simulink model "Path_Sim"  (R2018a)
settings: Solver=VariableStepAuto  StartTime=0.0  StopTime=10.0  RelTol=1e-3
libraries: dspindex x1
settings Model: Creator=chrros005  LastModifiedBy=chrros005

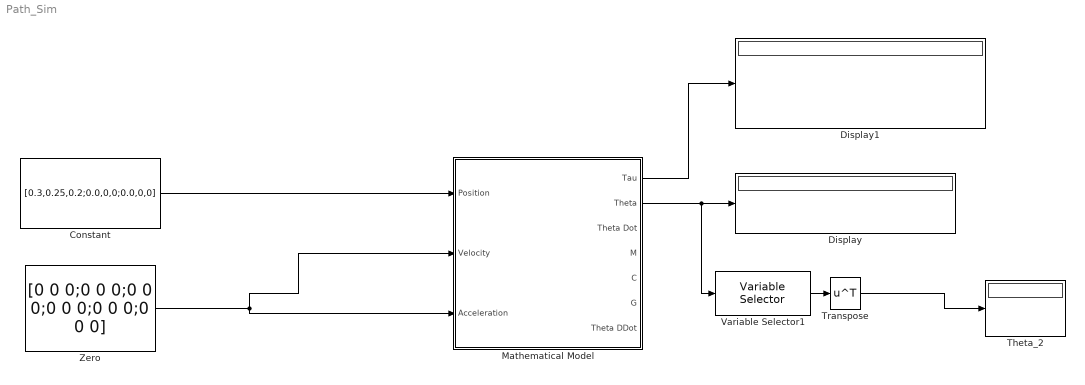
== system Path_Sim ==
  Constant : Constant  Value=[0.3,0.25,0.2;0.0,0,0;0.0,0,0]
  Display : Display
  Display1 : Display
  "Mathematical Model " : Subsystem  TreatAsAtomicUnit=on
  Theta_2 : Display
  Transpose : Math  Operator=transpose  SaturateOnIntegerOverflow=on
  Variable Selector1 : dspindex/Variable Selector  NumInputs=1  rowsOrCols=Rows  IdxMode=Fixed  Elements=2  ZerOneIdxMode=One-based  errmode=Clip Index  FillMode=on  FillValues=0
  Zero : Constant  Value=[0 0 0;0 0 0;0 0 0;0 0 0;0 0 0;0 0 0]
  wires:
  Constant/1 -> "Mathematical Model "/1(Position)
  Zero/1 -> "Mathematical Model "/2(Velocity), "Mathematical Model "/3(Acceleration)
  "Mathematical Model "/2(Theta) -> Variable Selector1/1, Display/1
  Variable Selector1/1 -> Transpose/1
  Transpose/1 -> Theta_2/1
  "Mathematical Model "/1(Tau) -> Display1/1

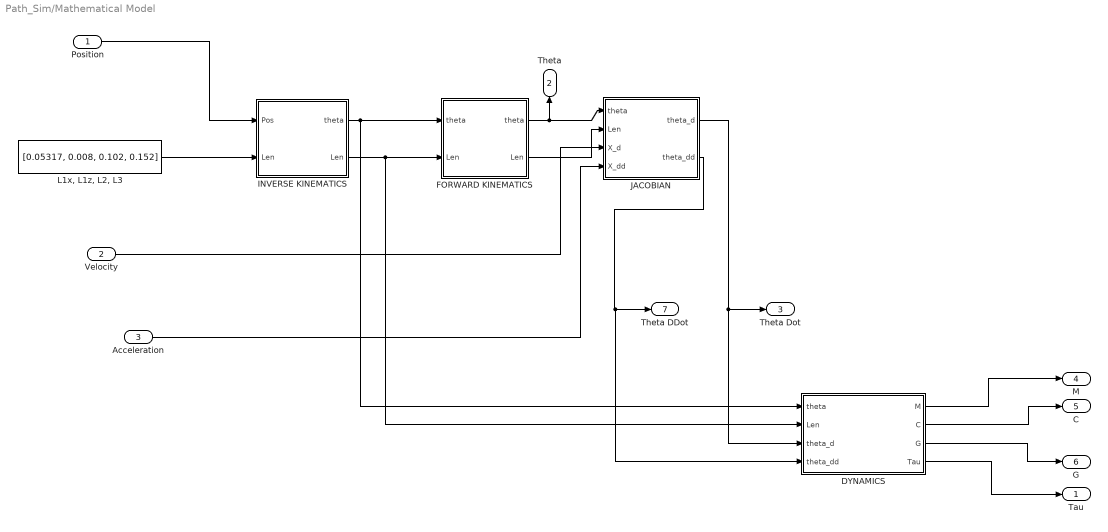
== system Path_Sim/Mathematical Model  ==
  Position : Inport
  Velocity : Inport  Port=2
  Acceleration : Inport  Port=3
  "DYNAMICS " : MATLAB Function  TreatAsAtomicUnit=on
  "FORWARD KINEMATICS " : MATLAB Function  TreatAsAtomicUnit=on
  "INVERSE KINEMATICS " : MATLAB Function  TreatAsAtomicUnit=on
  JACOBIAN : MATLAB Function  TreatAsAtomicUnit=on
  "L1x, L1z, L2, L3" : Constant  Value=[0.05317, 0.008, 0.102, 0.152]
  Tau : Outport
  Theta : Outport  Port=2
  Theta Dot : Outport  Port=3
  M : Outport  Port=4
  C : Outport  Port=5
  G : Outport  Port=6
  Theta DDot : Outport  Port=7
  wires:
  "INVERSE KINEMATICS "/1(theta) -> "FORWARD KINEMATICS "/1("theta "), "DYNAMICS "/1(theta)
  "FORWARD KINEMATICS "/2(Len) -> JACOBIAN/2(Len)
  "FORWARD KINEMATICS "/1(theta) -> JACOBIAN/1(theta), Theta/1
  JACOBIAN/2(theta_dd) -> Theta DDot/1, "DYNAMICS "/4(theta_dd)
  "L1x, L1z, L2, L3"/1 -> "INVERSE KINEMATICS "/2("Len ")
  "INVERSE KINEMATICS "/2(Len) -> "DYNAMICS "/2(Len), "FORWARD KINEMATICS "/2("Len ")
  "DYNAMICS "/4(Tau) -> Tau/1
  Acceleration/1 -> JACOBIAN/4(X_dd)
  Velocity/1 -> JACOBIAN/3(X_d)
  Position/1 -> "INVERSE KINEMATICS "/1(Pos)
  JACOBIAN/1(theta_d) -> Theta Dot/1, "DYNAMICS "/3(theta_d)
  "DYNAMICS "/1(M) -> M/1
  "DYNAMICS "/2(C) -> C/1
  "DYNAMICS "/3(G) -> G/1

== matlab function Path_Sim/Mathematical Model /FORWARD KINEMATICS  ==
  data: theta output; Len output; theta input; Len input
function [theta,Len]= FWD(theta, Len)
    
    s = size(theta);

    theta1 = theta(1,:);
    theta2 = theta(2,:);
    theta3 = theta(3,:);
   
    L1x = Len(1);
    L1z = Len(2);
    L2 = Len(3);
    L3 = Len(4); 
    

%     T = zeros(4,4,s(2));
%   
%     T = [ cos(theta2 + theta3)*cos(theta1), -sin(theta1), -sin(theta2 + theta3)*cos(theta1), cos(theta1)*(L1x + L3*cos(theta2 + theta3) + L2*cos(theta2));
%           cos(theta2 + theta3)*sin(theta1),  cos(theta1), -sin(theta2 + theta3)*sin(theta1), sin(theta1)*(L1x + L3*cos(theta2 + theta3) + L2*cos(theta2));
%                       sin(theta2 + theta3),            0,              cos(theta2 + theta3),               L1z + L3*sin(theta2 + theta3) + L2*sin(theta2);
%                                          0,            0,                                 0,                                                            1];

== matlab function Path_Sim/Mathematical Model /INVERSE KINEMATICS  ==
  data: Pos input; theta output; Len input; Len output
function [theta, Len] = INV(Pos, Len)

        s = size(Pos);

        x = zeros(1,s(2));
        y = zeros(1,s(2));
        z = zeros(1,s(2));

        theta1 = zeros(1,s(2));
        theta2 = zeros(1,s(2));
        theta3 = zeros(1,s(2));
        theta = zeros(3,s(2));
    
        x(:) = Pos(1,:);
        y(:) = Pos(2,:);
        z(:) = Pos(3,:);

        L1x = Len(1);
        L1z = Len(2);
        L2 = Len(3);
        L3 = Len(4);

        theta1(1,:) =  ( atan2(y(1,:),x(1,:)) );

        C3 = zeros(1,s(2));
        S3 = zeros(1,s(2));
        C3(1,:) = ( ( x(1,:) - L1x.*cos(theta1(1,:)) ).^2 + ( y(1,:) - L1x.*sin(theta1(1,:)) ).^2 + ( z(1,:) - L1z ).^2 - L2.^2 - L3.^2 )./( 2*L2*L3 );
        S3(1,:) = -sqrt(1 - C3(1,:).^2);

        theta2(1,:) =  ( atan2( z(1,:)-L1z, sqrt( (x(1,:)-L1x.*cos(theta1(1,:))).^2 + (y(1,:) - L1x.*sin(theta1(1,:))).^2 ) ) - atan2(L3.*S3(1,:), L2 + L3.*C3(1,:)) );

        theta3(1,:) =  ( atan2(S3(1,:), C3(1,:)) );

        theta = [theta1(1,:); theta2(1,:); theta3(1,:)];

== matlab function Path_Sim/Mathematical Model /JACOBIAN ==
  data: theta input; Len input; X_d input; theta_d output; theta_dd output; X_dd input
function [theta_d, theta_dd]= JAC(theta, Len, X_d, X_dd)

    s = size(theta);
    
    L1x = Len(1);
    L1z = Len(2);
    L2 = Len(3);
    L3 = Len(4);
        
    for i=1:s(2)

        theta1 = theta(1,i);
        theta2 = theta(2,i);
        theta3 = theta(3,i);
        
        J = zeros(6,3,s(2));

        J(:,:,i) = [-sin(theta1)*(L1x + L3*cos(theta2 + theta3) + L2*cos(theta2)), cos(theta1)*(L3*sin(theta2 + theta3) + L2*sin(theta2)), L3*sin(theta2 + theta3)*cos(theta1);
            cos(theta1)*(L1x + L3*cos(theta2 + theta3) + L2*cos(theta2)), sin(theta1)*(L3*sin(theta2 + theta3) + L2*sin(theta2)), L3*sin(theta2 + theta3)*sin(theta1);
                                                                 0,             - L3*cos(theta2 + theta3) - L2*cos(theta2),            -L3*cos(theta2 + theta3);
                                                                 0,                                           -sin(theta1),                        -sin(theta1);
                                                                 0,                                            cos(theta1),                         cos(theta1);
                                                                 1,                                                      0,                                   0]
        J_plus = zeros(3,6,s(2));
        J_plus(:,:,i) = [ -(2*sin(theta1)*(L1x + L3*cos(theta2 + theta3) + L2*cos(theta2)))/(L2^2*cos(2*theta2) + L3^2*cos(2*theta2 + 2*theta3) + L2^2 + L3^2 + 2*L1x^2 + 2*L2*L3*cos(2*theta2 + theta3) + 4*L3*L1x*cos(theta2 + theta3) + 2*L2*L3*cos(theta3) + 4*L2*L1x*cos(theta2) + 2), (2*cos(theta1)*(L1x + L3*cos(theta2 + theta3) + L2*cos(theta2)))/(L2^2*cos(2*theta2) + L3^2*cos(2*theta2 + 2*theta3) + L2^2 + L3^2 + 2*L1x^2 + 2*L2*L3*cos(2*theta2 + theta3) + 4*L3*L1x*cos(theta2 + theta3) + 2*L2*L3*cos(theta3) + 4*L2*L1x*cos(theta2) + 2),                                                                                                                                                                                 0,                                                                         0,                                                                        0, 1/((L2^2*cos(2*theta2))/2 + (L3^2*cos(2*theta2 + 2*theta3))/2 + L2^2/2 + L3^2/2 + L1x^2 + L2*L3*cos(2*theta2 + theta3) + 2*L3*L1x*cos(theta2 + theta3) + L2*L3*cos(theta3) + 2*L2*L1x*cos(theta2) + 1);
                                                                                                                                                         (cos(theta1)*(sin(theta2) - (L3^2*sin(theta2 + 2*theta3))/2 + (L3^2*sin(theta2))/2))/(L2*(L3^2 - L3^2*cos(theta3)^2 + 1)),                                                                                                                                       (sin(theta1)*(sin(theta2) - (L3^2*sin(theta2 + 2*theta3))/2 + (L3^2*sin(theta2))/2))/(L2*(L3^2 - L3^2*cos(theta3)^2 + 1)),                                                                            -(2*cos(theta2) - L3^2*cos(theta2 + 2*theta3) + L3^2*cos(theta2))/(L2*(L3^2 - L3^2*cos(2*theta3) + 2)),         (L3*cos(theta3)*sin(theta1))/(L2*(L3^2 - L3^2*cos(theta3)^2 + 1)),       -(L3*cos(theta1)*cos(theta3))/(L2*(L3^2 - L3^2*cos(theta3)^2 + 1)),                                                                                                                                                                                                      0;
                                                                                   (cos(theta1)*(L3^2*cos(theta3)^2*sin(theta2) - L3^2*sin(theta2) - sin(theta2) + L3^2*cos(theta2)*cos(theta3)*sin(theta3) + L2*L3*cos(theta2)*sin(theta3)))/(L2*(L3^2 - L3^2*cos(theta3)^2 + 1)),                                                                 (sin(theta1)*(L3^2*cos(theta3)^2*sin(theta2) - L3^2*sin(theta2) - sin(theta2) + L3^2*cos(theta2)*cos(theta3)*sin(theta3) + L2*L3*cos(theta2)*sin(theta3)))/(L2*(L3^2 - L3^2*cos(theta3)^2 + 1)), (cos(theta2) + L3^2*cos(theta2) - L3^2*cos(theta2)*cos(theta3)^2 + L3^2*cos(theta3)*sin(theta2)*sin(theta3) + L2*L3*sin(theta2)*sin(theta3))/(L2*(L3^2 - L3^2*cos(theta3)^2 + 1)), -(sin(theta1)*(L2 + L3*cos(theta3)))/(L2*(L3^2 - L3^2*cos(theta3)^2 + 1)), (cos(theta1)*(L2 + L3*cos(theta3)))/(L2*(L3^2 - L3^2*cos(theta3)^2 + 1)),                                                                                                                                                                                                      0];


        theta_d = zeros(3,s(2));
        theta_d(:,i) =  J_plus(:,:,i)*X_d(:,i); 
        theta1_d = theta_d(1,i);
        theta2_d = theta_d(2,i);
        theta3_d = theta_d(3,i);

        J_d = zeros(6,3,s(2));
        J_d(:,:,i) =   [   theta2_d*sin(theta1)*(L3*sin(theta2 + theta3) + L2*sin(theta2)) - theta1_d*cos(theta1)*(L1x + L3*cos(theta2 + theta3) + L2*cos(theta2)) + L3*theta3_d*sin(theta2 + theta3)*sin(theta1), theta2_d*cos(theta1)*(L3*cos(theta2 + theta3) + L2*cos(theta2)) - theta1_d*sin(theta1)*(L3*sin(theta2 + theta3) + L2*sin(theta2)) + L3*theta3_d*cos(theta2 + theta3)*cos(theta1), L3*theta2_d*cos(theta2 + theta3)*cos(theta1) + L3*theta3_d*cos(theta2 + theta3)*cos(theta1) - L3*theta1_d*sin(theta2 + theta3)*sin(theta1);
                 - theta2_d*cos(theta1)*(L3*sin(theta2 + theta3) + L2*sin(theta2)) - theta1_d*sin(theta1)*(L1x + L3*cos(theta2 + theta3) + L2*cos(theta2)) - L3*theta3_d*sin(theta2 + theta3)*cos(theta1), theta1_d*cos(theta1)*(L3*sin(theta2 + theta3) + L2*sin(theta2)) + theta2_d*sin(theta1)*(L3*cos(theta2 + theta3) + L2*cos(theta2)) + L3*theta3_d*cos(theta2 + theta3)*sin(theta1), L3*theta1_d*sin(theta2 + theta3)*cos(theta1) + L3*theta2_d*cos(theta2 + theta3)*sin(theta1) + L3*theta3_d*cos(theta2 + theta3)*sin(theta1);
                                                                                                                                                                                                        0,                                                                                           theta2_d*(L3*sin(theta2 + theta3) + L2*sin(theta2)) + L3*theta3_d*sin(theta2 + theta3),                                                                        L3*theta2_d*sin(theta2 + theta3) + L3*theta3_d*sin(theta2 + theta3);
                                                                                                                                                                                                        0,                                                                                                                                                            -theta1_d*cos(theta1),                                                                                                                      -theta1_d*cos(theta1);
                                                                                                                                                                                                        0,                                                                                                                                                            -theta1_d*sin(theta1),                                                                                                                      -theta1_d*sin(theta1);
                                                                                                                                                                                                 0,                                                                                                                                                                                0,                                                                                                                                          0];
                         %J_d ends here   
                         
        theta_dd = zeros(3,s(2));                 
        theta_dd(:,i) = J_plus(:,:,i)*( X_dd(:,i) - J_d(:,:,i)*theta_d(:,i) );
    end

== matlab function Path_Sim/Mathematical Model /DYNAMICS  ==
  data: theta input; Len input; M output; C output; G output; Tau output; theta_d input; theta_dd input
function [M,C,G,Tau]= DYN(theta, Len, theta_d,theta_dd)

    L1x = Len(1);
    L1z = Len(2);
    L2 = Len(3);
    L3 = Len(4)
      
    L1xc = L1x/2;
    L1zc = L1z/2;
    L2c = L2/2;
    L3c = L3/2;
    
    m = [0.14327;0.04977;0.15456];
    m1 = m(1);
    m2 = m(2);
    m3 = m(3);
    g = 9.80655 

    s = size(theta);
    
    for i=1:s(2)
        
        theta1 = theta(1,i);
        theta2 = theta(2,i);
        theta3 = theta(3,i);

        theta1_d = theta_d(1,i);
        theta2_d = theta_d(2,i);
        theta3_d = theta_d(3,i);

        M = zeros(3,3,s(2));
        M(:,:,i) = [ (L2c^2*m2)/2 + (L2c^2*m3)/2 + (L3c^2*m3)/2 + L1xc^2*m1 + L1xc^2*m2 + L1xc^2*m3 + (L2c^2*m2*cos(2*theta2))/2 + (L2c^2*m3*cos(2*theta2))/2 + (L3c^2*m3*cos(2*theta2 + 2*theta3))/2 + 2*L3c*L1xc*m3*cos(theta2 + theta3) + L2c*L3c*m3*cos(theta3) + 2*L2c*L1xc*m2*cos(theta2) + 2*L2c*L1xc*m3*cos(theta2) + L2c*L3c*m3*cos(2*theta2 + theta3) + 36456699500413941/36893488147419103232,                                                         0,                              0;
                                                                                                                                                                                                                                                                                                                                                                                               0, L2c^2*m2 + L2c^2*m3 + L3c^2*m3 + 2*L2c*L3c*m3*cos(theta3), L3c*m3*(L3c + L2c*cos(theta3));
                                                                                                                                                                                                                                                                                                                                                                                               0,                            L3c*m3*(L3c + L2c*cos(theta3)),                       L3c^2*m3];
        C = zeros(3,3,s(2));
        C(:,:,i) = [ - theta3_d*((L3c^2*m3*sin(2*theta2 + 2*theta3))/2 + L3c*L1xc*m3*sin(theta2 + theta3) + (L2c*L3c*m3*sin(theta3))/2 + (L2c*L3c*m3*sin(2*theta2 + theta3))/2) - theta2_d*((L2c^2*m2*sin(2*theta2))/2 + (L2c^2*m3*sin(2*theta2))/2 + (L3c^2*m3*sin(2*theta2 + 2*theta3))/2 + L3c*L1xc*m3*sin(theta2 + theta3) + L2c*L1xc*m2*sin(theta2) + L2c*L1xc*m3*sin(theta2) + L2c*L3c*m3*sin(2*theta2 + theta3)), -theta1_d*((L2c^2*m2*sin(2*theta2))/2 + (L2c^2*m3*sin(2*theta2))/2 + (L3c^2*m3*sin(2*theta2 + 2*theta3))/2 + L3c*L1xc*m3*sin(theta2 + theta3) + L2c*L1xc*m2*sin(theta2) + L2c*L1xc*m3*sin(theta2) + L2c*L3c*m3*sin(2*theta2 + theta3)), -theta1_d*((L3c^2*m3*sin(2*theta2 + 2*theta3))/2 + L3c*L1xc*m3*sin(theta2 + theta3) + (L2c*L3c*m3*sin(theta3))/2 + (L2c*L3c*m3*sin(2*theta2 + theta3))/2);
                                                                                                                                                                           theta1_d*((L2c^2*m2*sin(2*theta2))/2 + (L2c^2*m3*sin(2*theta2))/2 + (L3c^2*m3*sin(2*theta2 + 2*theta3))/2 + L3c*L1xc*m3*sin(theta2 + theta3) + L2c*L1xc*m2*sin(theta2) + L2c*L1xc*m3*sin(theta2) + L2c*L3c*m3*sin(2*theta2 + theta3)),                                                                                                                                                                                                       -L2c*L3c*m3*theta3_d*sin(theta3),                                                                                       - L2c*L3c*m3*theta2_d*sin(theta3) - L2c*L3c*m3*theta3_d*sin(theta3);
                                                                                                                                                                                                                                                        theta1_d*((L3c^2*m3*sin(2*theta2 + 2*theta3))/2 + L3c*L1xc*m3*sin(theta2 + theta3) + (L2c*L3c*m3*sin(theta3))/2 + (L2c*L3c*m3*sin(2*theta2 + theta3))/2),                                                                                                                                                                                                        L2c*L3c*m3*theta2_d*sin(theta3),                                                                                                                                                         0];
        G = zeros(3,1,s(2));
        G(:,:,i) = [ L2c*g*m2*cos(theta1);
                g*m3*(L3c*cos(theta2 + theta3) + L2*cos(theta2));
                L3c*g*m3*cos(theta2 + theta3)];

        Tau = zeros(3,s(2));    
        Tau(:,i) = M(:,:,i)*theta_dd(:,i) + C(:,:,i)*theta_d(:,i) + G(:,:,i);           
        
    end
